simulink model "LazoAbiertoYCerrado"  (Simulink 5.0)
settings: Solver=ode45  StartTime=0.0  StopTime=50  RelTol=1e-3
settings Model: LastModifiedBy=gaby

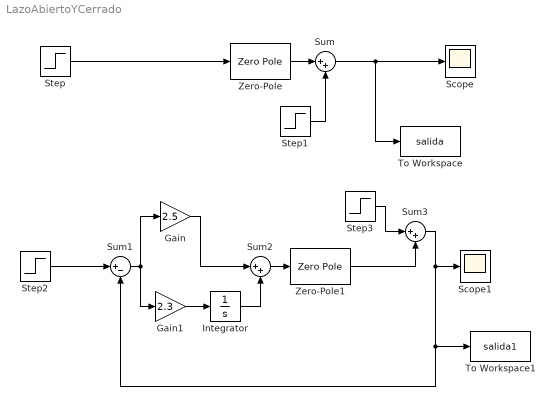
== system LazoAbiertoYCerrado ==
  Gain : Gain  Gain=2.5  SaturateOnIntegerOverflow=on
  Gain1 : Gain  Gain=2.3  SaturateOnIntegerOverflow=on
  Integrator : Integrator
  Scope : Scope
  Scope1 : Scope
  Step : Step  Time=0  After=2  SampleTime=0
  Step1 : Step  Time=20  SampleTime=0
  Step2 : Step  Time=0  After=2  SampleTime=0
  Step3 : Step  Time=20  SampleTime=0
  Sum : Sum  Inputs=|++  SaturateOnIntegerOverflow=on
  Sum1 : Sum  Inputs=|+-  SaturateOnIntegerOverflow=on
  Sum2 : Sum  Inputs=|++  SaturateOnIntegerOverflow=on
  Sum3 : Sum  Inputs=|++  SaturateOnIntegerOverflow=on
  To Workspace : ToWorkspace  VariableName=salida  SampleTime=-1  SaveFormat=Array
  To Workspace1 : ToWorkspace  VariableName=salida1  SampleTime=-1  SaveFormat=Array
  Zero-Pole : ZeroPole  Zeros=[]  Poles=[-2 -0.5]  Gain=[2.5]
  Zero-Pole1 : ZeroPole  Zeros=[]  Poles=[-2 -0.5]  Gain=[2.5]
  wires:
  Step2/1 -> Sum1/1
  Sum1/1 -> Gain/1, Gain1/1
  Gain/1 -> Sum2/1
  Integrator/1 -> Sum2/2
  Gain1/1 -> Integrator/1
  Sum2/1 -> Zero-Pole1/1
  Zero-Pole1/1 -> Sum3/2
  Step3/1 -> Sum3/1
  Sum3/1 -> Scope1/1, Sum1/2, To Workspace1/1
  Step/1 -> Zero-Pole/1
  Step1/1 -> Sum/2
  Zero-Pole/1 -> Sum/1
  Sum/1 -> Scope/1, To Workspace/1
